simulink subsystem "subrSinglePhaseMotor"  (R2024a)
settings: Solver=VariableStepAuto  StartTime=0.0  StopTime=10.0  RelTol=1e-3
model mask{RL=MOTR.RL, LL=MOTR.LL, KB=MOTR.KB, KT=MOTR.KT, J=MOTR.J, B=MOTR.B, D=MOTR.D}
  mask prompts: RL "Resistance"; LL "Inductance"; KB "Voltage Constant"; KT "Torque Constant"; J "Inertia"; B "Viscous Friction"; D "Coulomb Friction"
settings Model: Creator=anant  LastModifiedBy=anant

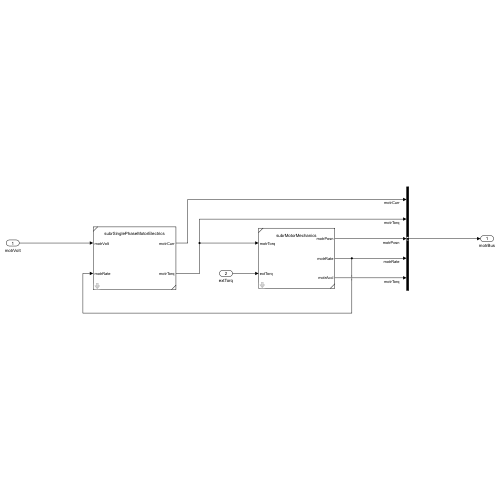
[thumbnail: Simulink's stored preview of the top-level diagram]
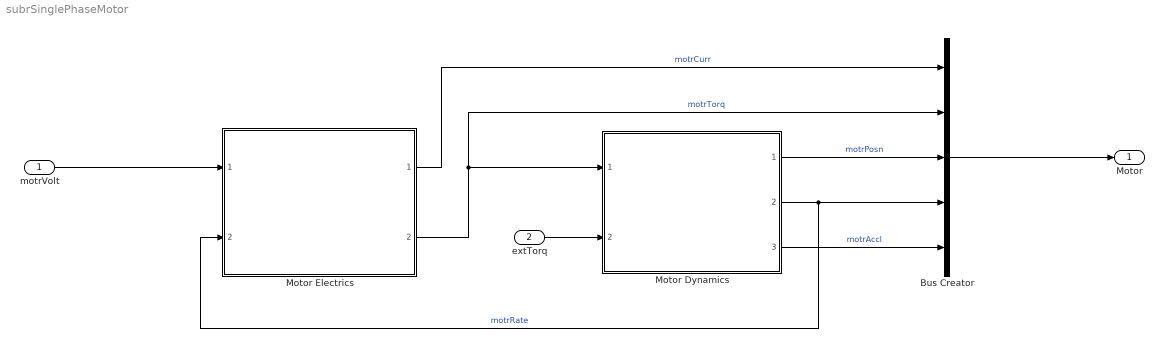
== system subrSinglePhaseMotor ==
  motrVolt : Inport
  extTorq : Inport  Port=2
  Bus Creator : BusCreator  Inputs=5
  Motor Dynamics : Subsystem  ReferencedSubsystem=subrMotorMechanics  J=J  B=B  D=D
  Motor Electrics : Subsystem  ReferencedSubsystem=subrSinglePhaseMotorElectrics  RL=RL  LL=LL  KB=KB  KT=KT
  Motor : Outport
  wires:
  Bus Creator/1 -> Motor/1
  Motor Dynamics/1 -> Bus Creator/3  "motrPosn"
  Motor Dynamics/3 -> Bus Creator/5  "motrAccl"
  Motor Dynamics/2 -> Bus Creator/4, Motor Electrics/2  "motrRate"
  Motor Electrics/2 -> Motor Dynamics/1, Bus Creator/2  "motrTorq"
  motrVolt/1 -> Motor Electrics/1
  extTorq/1 -> Motor Dynamics/2
  Motor Electrics/1 -> Bus Creator/1  "motrCurr"
